simulink model "MMS"  (R2017a)
settings: Solver=VariableStepAuto  StartTime=0.0  StopTime=30.0  RelTol=1e-3
settings Model: Creator=Michele  LastModifiedBy=Michele

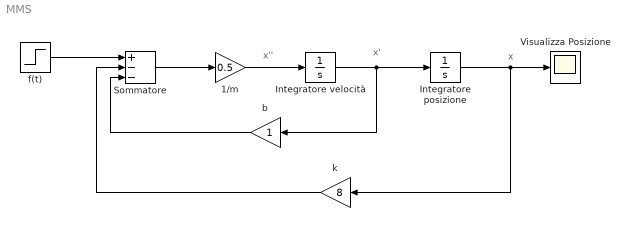
== system MMS ==
  note: x
  note: x'
  note: x''
  1/m : Gain  Gain=0.5
  Integratore posizione : Integrator
  Integratore velocità : Integrator
  Sommatore : Sum  Inputs=+--
  Visualizza Posizione : Scope
  b : Gain
  f(t) : Step  After=5  SampleTime=0
  k : Gain  Gain=8
  wires:
  f(t)/1 -> Sommatore/1
  Sommatore/1 -> 1/m/1
  1/m/1 -> Integratore velocità/1
  Integratore velocità/1 -> b/1, Integratore posizione/1
  Integratore posizione/1 -> k/1, Visualizza Posizione/1
  b/1 -> Sommatore/3
  k/1 -> Sommatore/2
